simulink model "Simulink"  (R2022b)
settings: Solver=ode4  StartTime=0.0  StopTime=1  FixedStep=0.0000010  RelTol=1e-3
values from neighbouring files (symbols this model uses):
  CFreq = 1080    [main.m]
  rr = 0.816    [main.m]
  rs = 0.435    [main.m]
  w_c = 2*pi*corner_frequency    (= 376.991118431)    [main.m]
libraries: simulink x1, spsRMSLib x1, eeGeneralControl x1, spspowerguiLib x1
settings Model: Creator=pouyaalaei  LastModifiedBy=igho
settings SolverCC: AlgebraicLoopSolver=TrustRegion
settings DebuggingCC: UnconnectedInputMsg=warning  UnconnectedOutputMsg=warning  UnconnectedLineMsg=warning  SFMachineParentedDataDiag=warning
settings ModelReferenceCC: EnableRefExpFcnMdlSchedulingChecks=on
settings RTWCC: DLArmComputeVersion=19.05

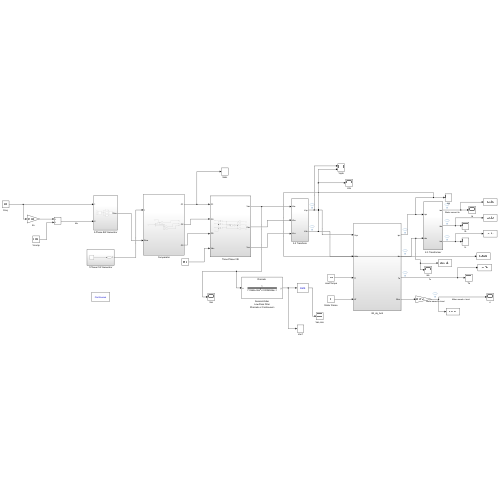
[thumbnail: Simulink's stored preview of the top-level diagram]
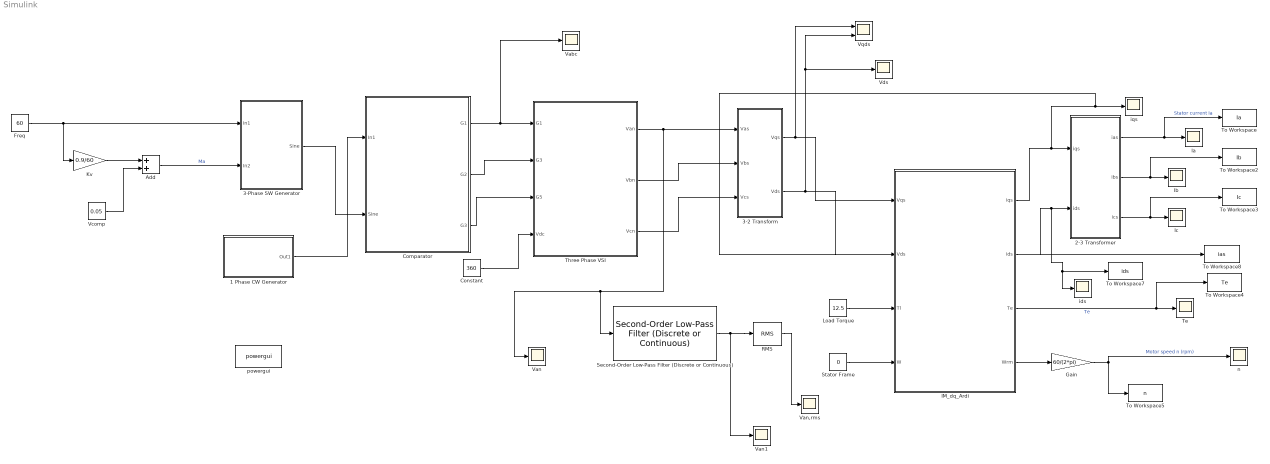
== system Simulink ==
  1 Phase CW Generator : Subsystem
  2-3 Transformer : Subsystem
  3-2 Transform : Subsystem
  3-Phase SW Generator : Subsystem
  Add : Sum
  Comparator : Subsystem
  Constant : Constant  Value=360
  Freq : Constant  Value=60
  Gain : Gain  Gain=60/(2*pi)
  IM_dq_Ardi : Subsystem
  Ia : Scope
  Ib : Scope
  Ic : Scope
  Kv : Gain  Gain=0.9/60
  Load Torque : Constant  Value=12.5
  RMS : spsRMSLib/RMS  TrueRMS=on  Freq=60  RMSInit=120  Ts=0
  Second-Order Low-Pass Filter (Discrete or Continuous) : eeGeneralControl/Second-Order Low-Pass Filter (Discrete or Continuous)  A1=1/w_c  A2=1/(w_c^2)  init_option=Inherited from block input  x0=0  Ts=-1
      settings: LibrarySourceBlock=|
      | ee_sl_lib/General Control/Second-Order
      | Low-Pass Filter
      | (Discrete or Continuous)
  Stator Frame : Constant  Value=0
  Te : Scope
  Three Phase VSI : Subsystem
  To Workspace : ToWorkspace  VariableName=Ia  SampleTime=-1
  To Workspace2 : ToWorkspace  VariableName=Ib  SampleTime=-1
  To Workspace3 : ToWorkspace  VariableName=Ic  SampleTime=-1
  To Workspace4 : ToWorkspace  VariableName=Te  SampleTime=-1
  To Workspace5 : ToWorkspace  VariableName=n  SampleTime=-1
  To Workspace7 : ToWorkspace  VariableName=ids  SampleTime=-1
  To Workspace8 : ToWorkspace  VariableName=ias  SampleTime=-1
  Vabc : Scope
  Van : Scope
  Van,rms : Scope
  Van1 : Scope
  Vcomp : Constant  Value=0.05
  Vds : Scope
  Vqds : Scope  NumInputPorts=2
  ids : Scope
  iqs : Scope
  n : Scope
  powergui : spspowerguiLib/powergui  Priority=1  SimulationMode=Continuous  SampleTime=50e-6  frequency=60  Iterations=50  frequencyindice=60  Pbase=100e6  ErrMax=1e-4  UnitsV=kV  UnitsW=MW  buscounter=0  FunctionMessages=off  echomessages=off  EnableUseOfTLC=off  CurrentSourceSwitches=off  DisableSnubberDevices=off  DisableRonSwitches=off  DisableVfSwitches=off  DisplayEquations=off  AutomaticDiscreteSolvers=off  SolverType=Tustin/Backward Euler (TBE)  Interpol=off  ExternalGateDelay=off  methode=off  Ts=100  x0status=blocks  SPID=on  SwTol=0  HookPort=off  NonlinearTolerance=1e-4  nMaxIteration=100  ContinueOnMaxIteration=off  RestoreLinks=warning  ResistiveCurrentMeasurement=off  Frange=[0:2:500]  Ylog=off  Xlog=on  ShowGrid=off  save=off  variable=ZData  structure=0  ZoomFFT=off  StartTime=0.0  cycles=1  DisplayStyle=1  fundamental=60  FreqAxis=off  MaxFrequency=1000  frequencyindicesteady=1  RmsSteady=1  display=off
  wires:
  Constant/1 -> Three Phase VSI/4(Vdc)
  Three Phase VSI/1(Van) -> Second-Order Low-Pass Filter (Discrete or Continuous)/1, Van/1, 3-2 Transform/1(Vas)
  Freq/1 -> 3-Phase SW Generator/1(In1), Kv/1
  1 Phase CW Generator/1(Out1) -> Comparator/1(In1)
  3-Phase SW Generator/1(Sine) -> Comparator/2(Sine)
  Comparator/1(G1) -> Vabc/1, Three Phase VSI/1(G1)
  Comparator/2(G2) -> Three Phase VSI/2(G3)
  Comparator/3(G3) -> Three Phase VSI/3(G5)
  2-3 Transformer/3(ics) -> Ic/1, To Workspace3/1
  IM_dq_Ardi/4(Wrm) -> Gain/1
  Gain/1 -> n/1, To Workspace5/1  "Motor speed n (rpm)"
  IM_dq_Ardi/3(Te) -> Te/1, To Workspace4/1  "Te"
  IM_dq_Ardi/2(ids) -> 2-3 Transformer/2(ids), ids/1, To Workspace7/1
  Stator Frame/1 -> IM_dq_Ardi/4(W)
  3-2 Transform/2(Vds) -> Vds/1, Vqds/2, IM_dq_Ardi/2(Vds)
  2-3 Transformer/1(ias) -> To Workspace/1, Ia/1  "Stator current Ia"
  IM_dq_Ardi/1(iqs) -> 2-3 Transformer/1(iqs), iqs/1, To Workspace8/1
  Three Phase VSI/2(Vbn) -> 3-2 Transform/2(Vbs)
  Load Torque/1 -> IM_dq_Ardi/3(Tl)
  3-2 Transform/1(Vqs) -> Vqds/1, IM_dq_Ardi/1(Vqs)
  Three Phase VSI/3(Vcn) -> 3-2 Transform/3(Vcs)
  2-3 Transformer/2(ibs) -> Ib/1, To Workspace2/1
  Second-Order Low-Pass Filter (Discrete or Continuous)/1 -> RMS/1, Van1/1
  RMS/1 -> Van,rms/1
  Add/1 -> 3-Phase SW Generator/2(In2)  "Ma"
  Kv/1 -> Add/1
  Vcomp/1 -> Add/2

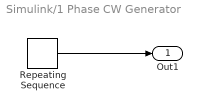
== system Simulink/1 Phase CW Generator ==
  Repeating Sequence : simulink/Sources/Repeating Sequence  rep_seq_t=[0 1/CFreq/4 3/CFreq/4 1/CFreq]  rep_seq_y=[0 1 -1 0]
  Out1 : Outport
  wires:
  Repeating Sequence/1 -> Out1/1

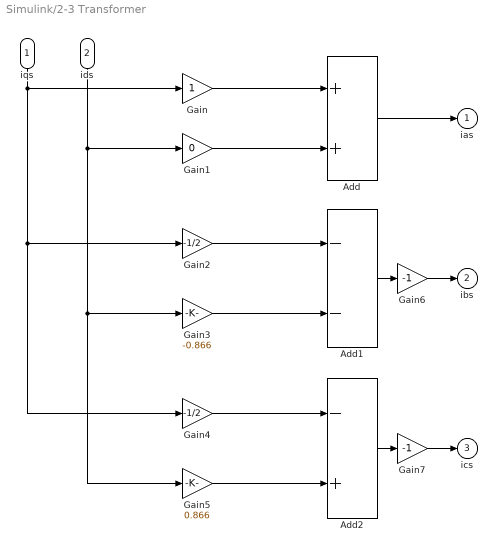
== system Simulink/2-3 Transformer ==
  iqs : Inport
  ids : Inport  Port=2
  Add : Sum
  Add1 : Sum  Inputs=--
  Add2 : Sum  Inputs=-+
  Gain : Gain
  Gain1 : Gain  Gain=0
  Gain2 : Gain  Gain=-1/2
  Gain3 : Gain  Gain=-0.866
  Gain4 : Gain  Gain=-1/2
  Gain5 : Gain  Gain=0.866
  Gain6 : Gain  Gain=-1
  Gain7 : Gain  Gain=-1
  ias : Outport  InitialOutput=0  VectorParamsAs1DForOutWhenUnconnected=off
  ibs : Outport  Port=2  InitialOutput=0  VectorParamsAs1DForOutWhenUnconnected=off
  ics : Outport  Port=3  InitialOutput=0  VectorParamsAs1DForOutWhenUnconnected=off
  wires:
  Gain/1 -> Add/1
  Gain1/1 -> Add/2
  Gain2/1 -> Add1/1
  Gain3/1 -> Add1/2
  Gain4/1 -> Add2/1
  Gain5/1 -> Add2/2
  Add2/1 -> Gain7/1
  Add1/1 -> Gain6/1
  Add/1 -> ias/1
  iqs/1 -> Gain/1, Gain2/1, Gain4/1
  ids/1 -> Gain1/1, Gain3/1, Gain5/1
  Gain6/1 -> ibs/1
  Gain7/1 -> ics/1

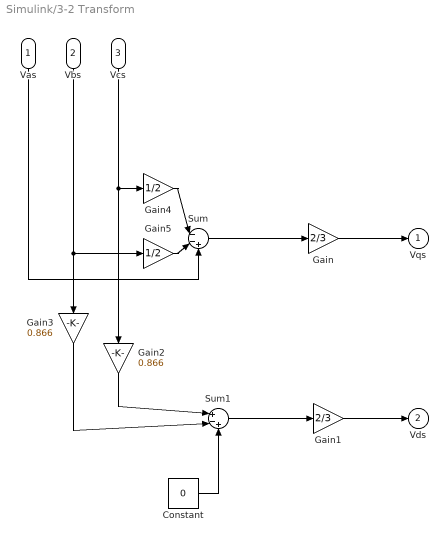
== system Simulink/3-2 Transform ==
  Vas : Inport
  Vbs : Inport  Port=2
  Vcs : Inport  Port=3
  Constant : Constant  Value=0
  Gain : Gain  Gain=2/3
  Gain1 : Gain  Gain=2/3
  Gain2 : Gain  Gain=0.866
  Gain3 : Gain  Gain=0.866
  Gain4 : Gain  Gain=1/2
  Gain5 : Gain  Gain=1/2
  Sum : Sum  Inputs=|--+
  Sum1 : Sum  Inputs=|+-+
  Vqs : Outport  InitialOutput=0  VectorParamsAs1DForOutWhenUnconnected=off
  Vds : Outport  Port=2  InitialOutput=0  VectorParamsAs1DForOutWhenUnconnected=off
  wires:
  Gain/1 -> Vqs/1
  Gain1/1 -> Vds/1
  Vas/1 -> Sum/3
  Vbs/1 -> Gain3/1, Gain5/1
  Sum/1 -> Gain/1
  Vcs/1 -> Gain2/1, Gain4/1
  Gain4/1 -> Sum/1
  Gain5/1 -> Sum/2
  Sum1/1 -> Gain1/1
  Gain2/1 -> Sum1/1
  Gain3/1 -> Sum1/2
  Constant/1 -> Sum1/3

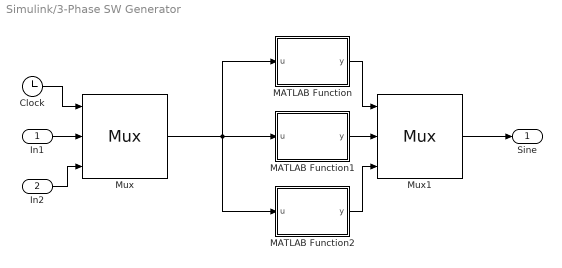
== system Simulink/3-Phase SW Generator ==
  In1 : Inport
  In2 : Inport  Port=2
  Clock : Clock
  MATLAB Function : MATLAB Function  TreatAsAtomicUnit=on
  MATLAB Function1 : MATLAB Function  TreatAsAtomicUnit=on
  MATLAB Function2 : MATLAB Function  TreatAsAtomicUnit=on
  Mux : Mux  Inputs=3
  Mux1 : Mux  Inputs=3
  Sine : Outport
  wires:
  Clock/1 -> Mux/1
  In1/1 -> Mux/2
  In2/1 -> Mux/3
  Mux/1 -> MATLAB Function/1(u), MATLAB Function2/1(u), MATLAB Function1/1(u)
  Mux1/1 -> Sine/1
  MATLAB Function/1(y) -> Mux1/1
  MATLAB Function2/1(y) -> Mux1/3
  MATLAB Function1/1(y) -> Mux1/2

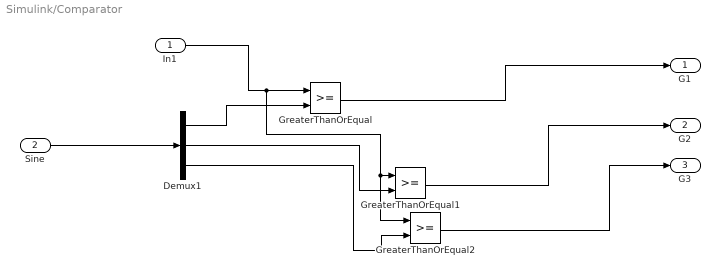
== system Simulink/Comparator ==
  In1 : Inport
  Sine : Inport  Port=2
  Demux1 : Demux  Outputs=3
  GreaterThanOrEqual : RelationalOperator  OutDataTypeStr=boolean  RndMeth=Simplest  InputSameDT=off
  GreaterThanOrEqual1 : RelationalOperator  OutDataTypeStr=boolean  RndMeth=Simplest  InputSameDT=off
  GreaterThanOrEqual2 : RelationalOperator  OutDataTypeStr=boolean  RndMeth=Simplest  InputSameDT=off
  G1 : Outport
  G2 : Outport  Port=2
  G3 : Outport  Port=3
  wires:
  In1/1 -> GreaterThanOrEqual1/1, GreaterThanOrEqual2/1, GreaterThanOrEqual/1
  Sine/1 -> Demux1/1
  GreaterThanOrEqual1/1 -> G2/1
  GreaterThanOrEqual2/1 -> G3/1
  Demux1/2 -> GreaterThanOrEqual1/2
  Demux1/1 -> GreaterThanOrEqual/2
  Demux1/3 -> GreaterThanOrEqual2/2
  GreaterThanOrEqual/1 -> G1/1

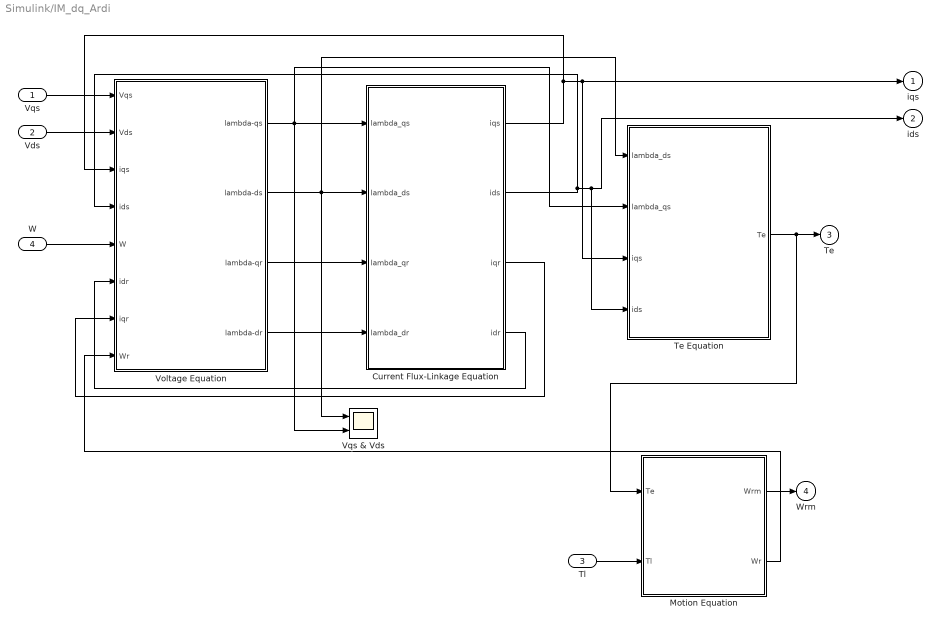
== system Simulink/IM_dq_Ardi ==
  Vqs : Inport
  Vds : Inport  Port=2
  Tl : Inport  Port=3
  W : Inport  Port=4
  Current Flux-Linkage Equation : Subsystem
  Motion Equation : Subsystem
  Te Equation : Subsystem
  Voltage Equation : Subsystem
  Vqs & Vds : Scope  NumInputPorts=2
  iqs : Outport  InitialOutput=0  VectorParamsAs1DForOutWhenUnconnected=off
  ids : Outport  Port=2  InitialOutput=0  VectorParamsAs1DForOutWhenUnconnected=off
  Te : Outport  Port=3  InitialOutput=0  VectorParamsAs1DForOutWhenUnconnected=off
  Wrm : Outport  Port=4  InitialOutput=0  VectorParamsAs1DForOutWhenUnconnected=off
  wires:
  Vqs/1 -> Voltage Equation/1(Vqs)
  Vds/1 -> Voltage Equation/2(Vds)
  Tl/1 -> Motion Equation/2(Tl)
  W/1 -> Voltage Equation/5(W)
  Te Equation/1(Te) -> Te/1, Motion Equation/1(Te)
  Current Flux-Linkage Equation/1(iqs) -> Voltage Equation/3(iqs), iqs/1, Te Equation/3(iqs)
  Current Flux-Linkage Equation/2(ids) -> Voltage Equation/4(ids), ids/1, Te Equation/4(ids)
  Current Flux-Linkage Equation/3(iqr) -> Voltage Equation/7(iqr)
  Voltage Equation/1(lambda-qs) -> Vqs & Vds/2, Current Flux-Linkage Equation/1(lambda_qs), Te Equation/2(lambda_qs)
  Voltage Equation/2(lambda-ds) -> Te Equation/1(lambda_ds), Vqs & Vds/1, Current Flux-Linkage Equation/2(lambda_ds)
  Voltage Equation/3(lambda-qr) -> Current Flux-Linkage Equation/3(lambda_qr)
  Voltage Equation/4(lambda-dr) -> Current Flux-Linkage Equation/4(lambda_dr)
  Current Flux-Linkage Equation/4(idr) -> Voltage Equation/6(idr)
  Motion Equation/2(Wr) -> Voltage Equation/8(Wr)
  Motion Equation/1(Wrm) -> Wrm/1

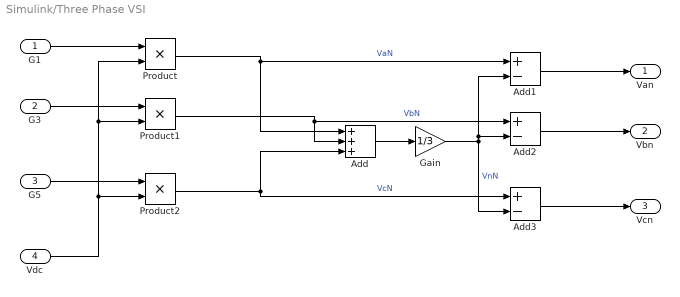
== system Simulink/Three Phase VSI ==
  G1 : Inport
  G3 : Inport  Port=2
  G5 : Inport  Port=3
  Vdc : Inport  Port=4
  Add : Sum  Inputs=+++
  Add1 : Sum  Inputs=+-
  Add2 : Sum  Inputs=+-
  Add3 : Sum  Inputs=+-
  Gain : Gain  Gain=1/3
  Product : Product
  Product1 : Product
  Product2 : Product
  Van : Outport
  Vbn : Outport  Port=2
  Vcn : Outport  Port=3
  wires:
  G3/1 -> Product1/1
  G1/1 -> Product/1
  G5/1 -> Product2/1
  Vdc/1 -> Product/2, Product1/2, Product2/2
  Product/1 -> Add1/1, Add/1  "VaN"
  Product1/1 -> Add2/1, Add/2  "VbN"
  Product2/1 -> Add/3, Add3/1  "VcN"
  Add/1 -> Gain/1
  Gain/1 -> Add1/2, Add2/2, Add3/2  "VnN"
  Add1/1 -> Van/1
  Add2/1 -> Vbn/1
  Add3/1 -> Vcn/1

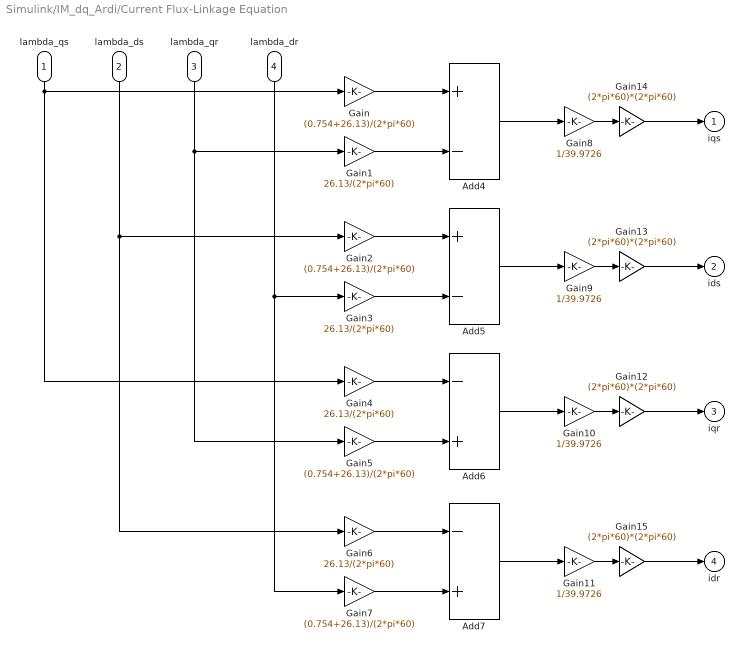
== system Simulink/IM_dq_Ardi/Current Flux-Linkage Equation ==
  lambda_qs : Inport
  lambda_ds : Inport  Port=2
  lambda_qr : Inport  Port=3
  lambda_dr : Inport  Port=4
  Add4 : Sum  Inputs=+-
  Add5 : Sum  Inputs=+-
  Add6 : Sum  Inputs=-+
  Add7 : Sum  Inputs=-+
  Gain{,2,5,7} (4 alike) : Gain  Gain=(0.754+26.13)/(2*pi*60)
  Gain{1,3..4,6} (4 alike) : Gain  Gain=26.13/(2*pi*60)
  Gain{8..11} (4 alike) : Gain  Gain=1/39.9726
  Gain{12..15} (4 alike) : Gain  Gain=(2*pi*60)*(2*pi*60)
  iqs : Outport  InitialOutput=0  VectorParamsAs1DForOutWhenUnconnected=off
  ids : Outport  Port=2  InitialOutput=0  VectorParamsAs1DForOutWhenUnconnected=off
  iqr : Outport  Port=3  InitialOutput=0  VectorParamsAs1DForOutWhenUnconnected=off
  idr : Outport  Port=4  InitialOutput=0  VectorParamsAs1DForOutWhenUnconnected=off
  wires:
  Gain1/1 -> Add4/2
  Gain/1 -> Add4/1
  Gain2/1 -> Add5/1
  Gain3/1 -> Add5/2
  Gain4/1 -> Add6/1
  Gain5/1 -> Add6/2
  Gain6/1 -> Add7/1
  Gain7/1 -> Add7/2
  Add4/1 -> Gain8/1
  Add5/1 -> Gain9/1
  Add6/1 -> Gain10/1
  Add7/1 -> Gain11/1
  lambda_qs/1 -> Gain/1, Gain4/1
  lambda_qr/1 -> Gain1/1, Gain5/1
  Gain10/1 -> Gain12/1
  Gain9/1 -> Gain13/1
  Gain8/1 -> Gain14/1
  Gain11/1 -> Gain15/1
  lambda_ds/1 -> Gain2/1, Gain6/1
  lambda_dr/1 -> Gain3/1, Gain7/1
  Gain14/1 -> iqs/1
  Gain13/1 -> ids/1
  Gain12/1 -> iqr/1
  Gain15/1 -> idr/1

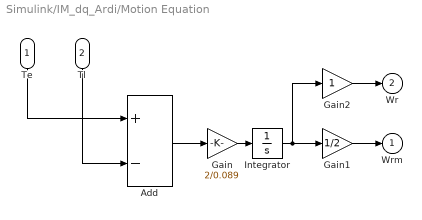
== system Simulink/IM_dq_Ardi/Motion Equation ==
  Te : Inport
  Tl : Inport  Port=2
  Add : Sum  Inputs=+-
  Gain : Gain  Gain=2/0.089
  Gain1 : Gain  Gain=1/2
  Gain2 : Gain
  Integrator : Integrator
  Wrm : Outport  InitialOutput=0  VectorParamsAs1DForOutWhenUnconnected=off
  Wr : Outport  Port=2  InitialOutput=0  VectorParamsAs1DForOutWhenUnconnected=off
  wires:
  Te/1 -> Add/1
  Tl/1 -> Add/2
  Gain/1 -> Integrator/1
  Add/1 -> Gain/1
  Integrator/1 -> Gain2/1, Gain1/1
  Gain2/1 -> Wr/1
  Gain1/1 -> Wrm/1

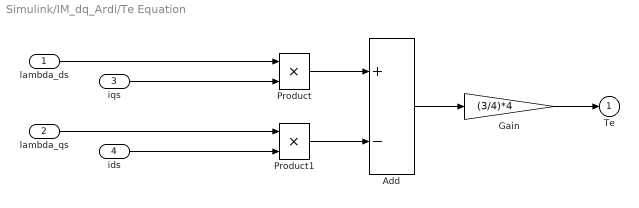
== system Simulink/IM_dq_Ardi/Te Equation ==
  lambda_ds : Inport
  lambda_qs : Inport  Port=2
  iqs : Inport  Port=3
  ids : Inport  Port=4
  Add : Sum  Inputs=+-
  Gain : Gain  Gain=(3/4)*4
  Product : Product  RndMeth=Zero
  Product1 : Product  RndMeth=Zero
  Te : Outport  InitialOutput=0  VectorParamsAs1DForOutWhenUnconnected=off
  wires:
  Gain/1 -> Te/1
  Add/1 -> Gain/1
  lambda_ds/1 -> Product/1
  iqs/1 -> Product/2
  lambda_qs/1 -> Product1/1
  ids/1 -> Product1/2
  Product/1 -> Add/1
  Product1/1 -> Add/2

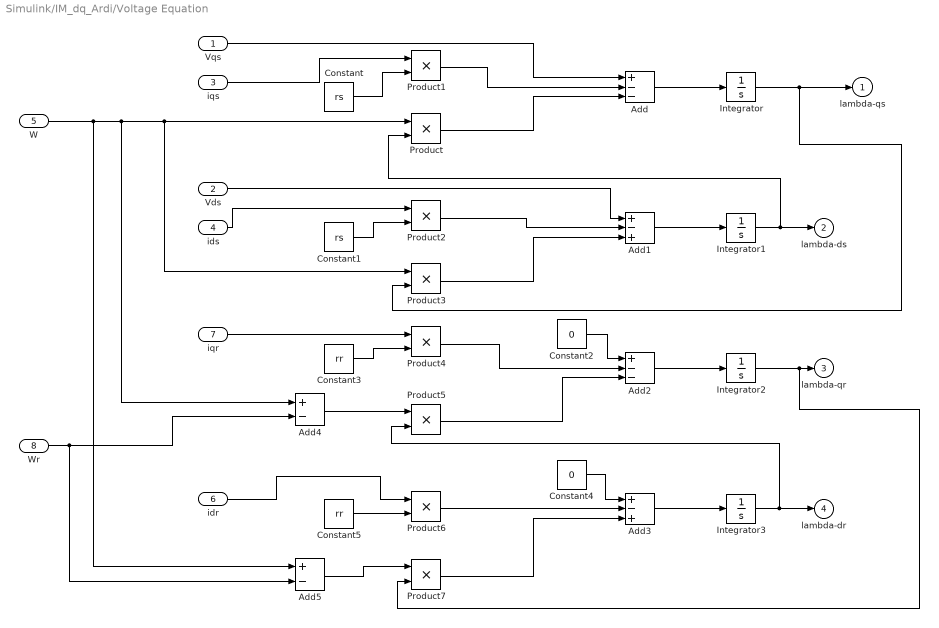
== system Simulink/IM_dq_Ardi/Voltage Equation ==
  Vqs : Inport
  Vds : Inport  Port=2
  iqs : Inport  Port=3
  ids : Inport  Port=4
  W : Inport  Port=5
  idr : Inport  Port=6
  iqr : Inport  Port=7
  Wr : Inport  Port=8
  Add : Sum  Inputs=+--
  Add1 : Sum  Inputs=+-+
  Add2 : Sum  Inputs=+--
  Add3 : Sum  Inputs=+-+
  Add4 : Sum  Inputs=+-
  Add5 : Sum  Inputs=+-
  Constant : Constant  Value=rs
  Constant1 : Constant  Value=rs
  Constant2 : Constant  Value=0
  Constant3 : Constant  Value=rr
  Constant4 : Constant  Value=0
  Constant5 : Constant  Value=rr
  Integrator{,1..3} (4 alike) : Integrator
  Product{,1..7} (8 alike) : Product
  lambda-qs : Outport  InitialOutput=0  VectorParamsAs1DForOutWhenUnconnected=off
  lambda-ds : Outport  Port=2  InitialOutput=0  VectorParamsAs1DForOutWhenUnconnected=off
  lambda-qr : Outport  Port=3  InitialOutput=0  VectorParamsAs1DForOutWhenUnconnected=off
  lambda-dr : Outport  Port=4  InitialOutput=0  VectorParamsAs1DForOutWhenUnconnected=off
  wires:
  Integrator/1 -> Product3/2, lambda-qs/1
  Integrator1/1 -> Product/2, lambda-ds/1
  Integrator2/1 -> Product7/2, lambda-qr/1
  Integrator3/1 -> Product5/2, lambda-dr/1
  Vqs/1 -> Add/1
  iqs/1 -> Product1/1
  Constant/1 -> Product1/2
  Add/1 -> Integrator/1
  Product1/1 -> Add/2
  Product/1 -> Add/3
  Vds/1 -> Add1/1
  ids/1 -> Product2/1
  Constant1/1 -> Product2/2
  Product2/1 -> Add1/2
  Add1/1 -> Integrator1/1
  Add2/1 -> Integrator2/1
  Add3/1 -> Integrator3/1
  Product3/1 -> Add1/3
  Constant2/1 -> Add2/1
  Constant3/1 -> Product4/2
  iqr/1 -> Product4/1
  Product4/1 -> Add2/2
  Wr/1 -> Add5/2, Add4/2
  W/1 -> Add5/1, Add4/1, Product3/1, Product/1
  Add4/1 -> Product5/1
  Product5/1 -> Add2/3
  Constant4/1 -> Add3/1
  Constant5/1 -> Product6/2
  idr/1 -> Product6/1
  Product6/1 -> Add3/2
  Add5/1 -> Product7/1
  Product7/1 -> Add3/3

== matlab function Simulink/3-Phase SW Generator/MATLAB Function ==
  data: u input; y output
function y = fcn(u)


y = u(3)*sin(2*pi*u(2)*u(1));

== matlab function Simulink/3-Phase SW Generator/MATLAB Function2 ==
  data: u input; y output
function y = fcn(u)

y = u(3)*sin(2*pi*u(2)*u(1)+(2*pi/3));

== matlab function Simulink/3-Phase SW Generator/MATLAB Function1 ==
  data: u input; y output
function y = fcn(u)

y = u(3)*sin(2*pi*u(2)*u(1)-(2*pi/3));
